simulink model "MotorControllerSimulation"  (R2016a)
settings: Solver=VariableStepAuto  StartTime=0.0  StopTime=simTime  RelTol=1e-3
values from neighbouring files (symbols this model uses):
  currentSensorResistance = 0.001    [Initialize.m]
  D_Current = 0    [Initialize.m]
  D_Velocity = 0    [Initialize.m]
  dampingCoefficient = 0    [Initialize.m]
  driverResistance = 1    [Initialize.m]
  gm = 1 / 0.0013    (= 769.230769231)    [Initialize.m]
  I_Current = 1    [Initialize.m]
  I_Velocity = 1    [Initialize.m]
  maxCurrent = 30    [Initialize.m]
  maxVelocity = 1000    [Initialize.m]
  mosfetGateResistance = 1    [Initialize.m]
  motorResistance = 1    [Initialize.m]
  P_Current = 1    [Initialize.m]
  P_Velocity = 1    [Initialize.m]
  sampleRate = 1000    [Initialize.m]
  switchingPeriod = 1/switchingFrequency    (= 0.0002)    [Initialize.m]
  targetVelocity = 300    [Initialize.m]
  torqueConstant = 1    [Initialize.m]
libraries: fl_lib x25, nesl_utility x5, simulink x4
settings Model: Creator=Koltin Kosik-Harvey  LastModifiedBy=Koltin Kosik-Harvey

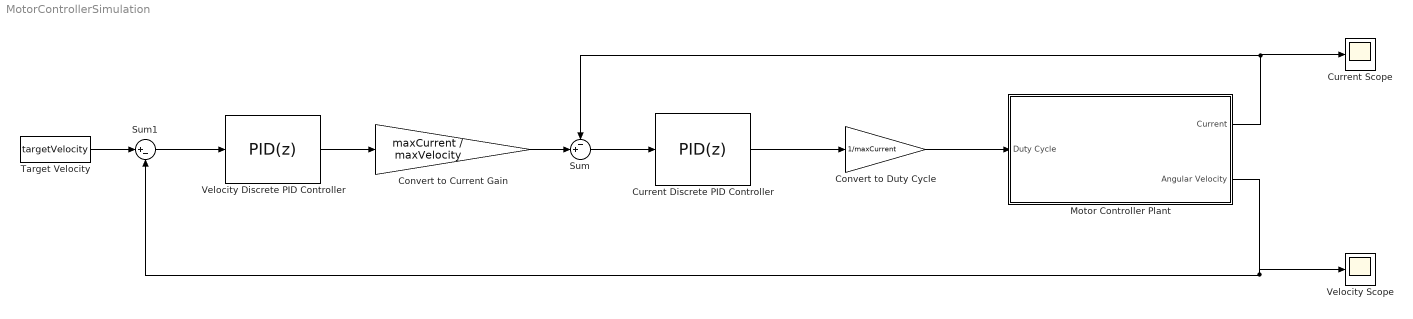
== system MotorControllerSimulation ==
  Convert to Current Gain : Gain  Gain=maxCurrent / maxVelocity
  Convert to Duty Cycle : Gain  Gain=1/maxCurrent
  Current Discrete PID Controller : simulink/Continuous/PID Controller  Controller=PID  TimeDomain=Discrete-time  SampleTime=sampleRate  IntegratorMethod=Forward Euler  FilterMethod=Forward Euler  Form=Parallel  UseFilter=on  ControllerParametersSource=internal  P=P_Current  I=I_Current  D=D_Current  N=100  InitialConditionSource=internal  InitialConditionForIntegrator=0  InitialConditionForFilter=0  ExternalReset=none  LimitOutput=on  UpperSaturationLimit=maxCurrent  LowerSaturationLimit=0  LinearizeAsGain=off  AntiWindupMode=none  Kb=1  TrackingMode=off  Kt=1  PParamMin=[]  PParamMax=[]  IParamMin=[]  IParamMax=[]  DParamMin=[]  DParamMax=[]  NParamMin=[]  NParamMax=[]  KbParamMin=[]  KbParamMax=[]  KtParamMin=[]  KtParamMax=[]  POutMin=[]  POutMax=[]  IOutMin=[]  IOutMax=[]  DOutMin=[]  DOutMax=[]  NOutMin=[]  NOutMax=[]  KbOutMin=[]  KbOutMax=[]  KtOutMin=[]  KtOutMax=[]  IntegratorOutMin=[]  IntegratorOutMax=[]  FilterOutMin=[]  FilterOutMax=[]  SumOutMin=[]  SumOutMax=[]  SumI1OutMin=[]  SumI1OutMax=[]  SumI2OutMin=[]  SumI2OutMax=[]  SumI3OutMin=[]  SumI3OutMax=[]  SumDOutMin=[]  SumDOutMax=[]  SaturationOutMin=[]  SaturationOutMax=[]  IntegratorContinuousStateAttributes=''  IntegratorStateMustResolveToSignalObject=off  IntegratorRTWStateStorageClass=Auto  FilterContinuousStateAttributes=''  FilterStateMustResolveToSignalObject=off  FilterRTWStateStorageClass=Auto  DifferentiatorICPrevScaledInput=0  DifferentiatorOutMin=[]  DifferentiatorOutMax=[]
  Current Scope : Scope
  Motor Controller Plant : Subsystem
  Sum : Sum  Inputs=-+|
  Sum1 : Sum  Inputs=|+-
  Target Velocity : Constant  Value=targetVelocity
  Velocity Discrete PID Controller : simulink/Continuous/PID Controller  Controller=PID  TimeDomain=Discrete-time  SampleTime=sampleRate  IntegratorMethod=Forward Euler  FilterMethod=Forward Euler  Form=Parallel  UseFilter=on  ControllerParametersSource=internal  P=P_Velocity  I=I_Velocity  D=D_Velocity  N=100  InitialConditionSource=internal  InitialConditionForIntegrator=0  InitialConditionForFilter=0  ExternalReset=none  LimitOutput=on  UpperSaturationLimit=maxVelocity  LowerSaturationLimit=0  LinearizeAsGain=off  AntiWindupMode=none  Kb=1  TrackingMode=off  Kt=1  PParamMin=[]  PParamMax=[]  IParamMin=[]  IParamMax=[]  DParamMin=[]  DParamMax=[]  NParamMin=[]  NParamMax=[]  KbParamMin=[]  KbParamMax=[]  KtParamMin=[]  KtParamMax=[]  POutMin=[]  POutMax=[]  IOutMin=[]  IOutMax=[]  DOutMin=[]  DOutMax=[]  NOutMin=[]  NOutMax=[]  KbOutMin=[]  KbOutMax=[]  KtOutMin=[]  KtOutMax=[]  IntegratorOutMin=[]  IntegratorOutMax=[]  FilterOutMin=[]  FilterOutMax=[]  SumOutMin=[]  SumOutMax=[]  SumI1OutMin=[]  SumI1OutMax=[]  SumI2OutMin=[]  SumI2OutMax=[]  SumI3OutMin=[]  SumI3OutMax=[]  SumDOutMin=[]  SumDOutMax=[]  SaturationOutMin=[]  SaturationOutMax=[]  IntegratorContinuousStateAttributes=''  IntegratorStateMustResolveToSignalObject=off  IntegratorRTWStateStorageClass=Auto  FilterContinuousStateAttributes=''  FilterStateMustResolveToSignalObject=off  FilterRTWStateStorageClass=Auto  DifferentiatorICPrevScaledInput=0  DifferentiatorOutMin=[]  DifferentiatorOutMax=[]
  Velocity Scope : Scope
  wires:
  Velocity Discrete PID Controller/1 -> Convert to Current Gain/1
  Current Discrete PID Controller/1 -> Convert to Duty Cycle/1
  Convert to Duty Cycle/1 -> Motor Controller Plant/1(Duty Cycle)
  Motor Controller Plant/1("Current ") -> Current Scope/1, Sum/1
  Convert to Current Gain/1 -> Sum/2
  Sum/1 -> Current Discrete PID Controller/1
  Motor Controller Plant/2(Angular Velocity) -> Sum1/2, Velocity Scope/1
  Target Velocity/1 -> Sum1/1
  Sum1/1 -> Velocity Discrete PID Controller/1

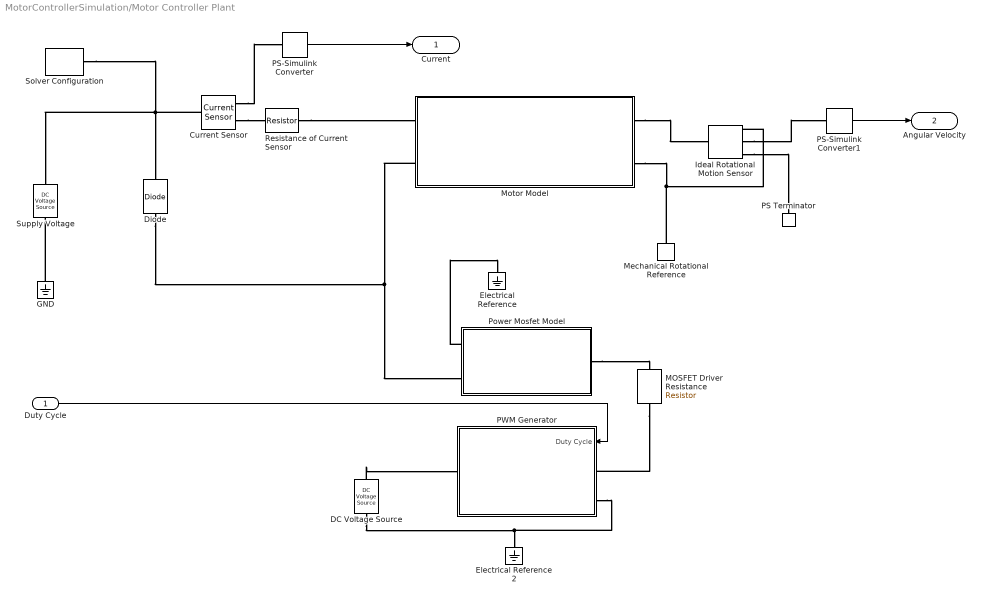
== system MotorControllerSimulation/Motor Controller Plant ==
  Duty Cycle : Inport
  Current Sensor : fl_lib/Electrical/Electrical Sensors/Current Sensor
  DC Voltage Source : fl_lib/Electrical/Electrical Sources/DC Voltage Source  v0=gateVoltage V
  Diode : fl_lib/Electrical/Electrical Elements/Diode  Vf=0.03 V  Ron=0.0001 Ohm  Goff=1e-8 1/Ohm  i_specify=off  i_priority=None  i=0 A  v_specify=off  v_priority=None  v=0 V
  Electrical Reference : fl_lib/Electrical/Electrical Elements/Electrical Reference
  Electrical Reference 2 : fl_lib/Electrical/Electrical Elements/Electrical Reference
  GND : fl_lib/Electrical/Electrical Elements/Electrical Reference
  Ideal Rotational Motion Sensor : fl_lib/Mechanical/Mechanical Sensors/Ideal Rotational Motion Sensor  offset=0 rad
  MOSFET Driver Resistance : fl_lib/Electrical/Electrical Elements/Resistor  R=driverResistance Ohm  i_specify=off  i_priority=None  i=0 A  v_specify=off  v_priority=None  v=0 V
  Mechanical Rotational Reference : fl_lib/Mechanical/Rotational Elements/Mechanical Rotational Reference
  Motor Model : Subsystem
  PS Terminator : fl_lib/Physical Signals/Sinks/PS Terminator
  PS-Simulink Converter : nesl_utility/PS-Simulink Converter  PhysicalDomain=network_engine_domain  SubClassName=ps_output  LeftPortType=input  RightPortType=output  PseudoPeriodic=off  Frequencies=[]  Unit=1  AffineConversion=off
  PS-Simulink Converter1 : nesl_utility/PS-Simulink Converter  PhysicalDomain=network_engine_domain  SubClassName=ps_output  LeftPortType=input  RightPortType=output  PseudoPeriodic=off  Frequencies=[]  Unit=1  AffineConversion=off
  PWM Generator : Subsystem
  Power Mosfet Model : Subsystem
  "Resistance of Current Sensor " : fl_lib/Electrical/Electrical Elements/Resistor  R=currentSensorResistance Ohm  i_specify=off  i_priority=None  i=0 A  v_specify=off  v_priority=None  v=0 V
  Solver Configuration : nesl_utility/Solver Configuration  PhysicalDomain=network_engine_domain  SubClassName=solver  LeftPortType=input  RightPortType=generic  Accelerate=off  Tones=[]  Harmonics=[]  SimulateNoise=off  Profile=off  UseLocalSampling=off  EnableSwitchedLinearOptims=on  FrequencyDomain=off  UseCCode=off  RelTol=0.001  AbsTol=1e-06  MinStep=1e-09  ToWorkspace=off  RevertToSquareIcSolve=off  NumHomotopyIterations=100  PhasorMode=off  PhasorModeNumHarmonics=1  OverrideAbsTol=off  DoDC=off  ResidualTolerance=1e-09  UseLocalSolver=off  LocalSolverChoice=NE_BACKWARD_EULER_ADVANCER  LocalSolverSampleTime=0.001  DoFixedCost=off  MaxNonlinIter=3  MaxModeIter=2  LinearAlgebra=Sparse  DelaysMemoryBudget=1024  AutomaticFiltering=on  FilteringTimeConstant=0.001
  Supply Voltage : fl_lib/Electrical/Electrical Sources/DC Voltage Source  v0=supplyVoltage V
  "Current " : Outport
  Angular Velocity : Outport  Port=2
  wires:
  Duty Cycle/1 -> PWM Generator/1(Duty Cycle)
  PS-Simulink Converter/1 -> "Current "/1
  PS-Simulink Converter1/1 -> Angular Velocity/1
  connections:
  DC Voltage Source/LConn1 -- PWM Generator/RConn1
  Power Mosfet Model/LConn1 -- MOSFET Driver Resistance/RConn1
  PWM Generator/LConn2 -- DC Voltage Source/RConn1 -- Electrical Reference 2/LConn1
  Current Sensor/RConn2 -- "Resistance of Current Sensor "/LConn1
  "Resistance of Current Sensor "/RConn1 -- Motor Model/LConn1
  Ideal Rotational Motion Sensor/RConn2 -- PS-Simulink Converter1/LConn1
  Power Mosfet Model/RConn1 -- Electrical Reference/LConn1
  Motor Model/RConn1 -- Ideal Rotational Motion Sensor/LConn1
  Current Sensor/RConn1 -- PS-Simulink Converter/LConn1
  Ideal Rotational Motion Sensor/RConn3 -- PS Terminator/LConn1
  Motor Model/LConn2 -- Diode/LConn1 -- Power Mosfet Model/RConn2
  Motor Model/RConn2 -- Ideal Rotational Motion Sensor/RConn1 -- Mechanical Rotational Reference/LConn1
  Current Sensor/LConn1 -- Solver Configuration/RConn1 -- Supply Voltage/LConn1 -- Diode/RConn1
  MOSFET Driver Resistance/LConn1 -- PWM Generator/LConn1
  GND/LConn1 -- Supply Voltage/RConn1

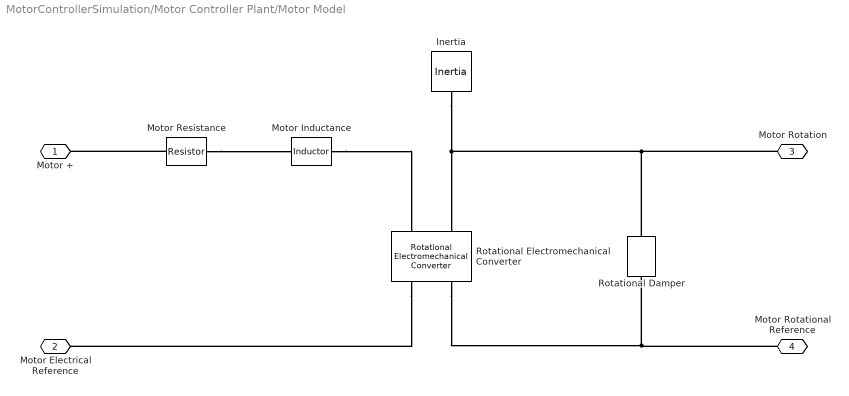
== system MotorControllerSimulation/Motor Controller Plant/Motor Model ==
  Inertia : fl_lib/Mechanical/Rotational Elements/Inertia  inertia=motorInertia kg*m^2  w_specify=off  w_priority=High  w=0 rad/s  t_specify=off  t_priority=None  t=0 N*m
  Motor Resistance : fl_lib/Electrical/Electrical Elements/Resistor  R=motorResistance Ohm  i_specify=off  i_priority=None  i=0 A  v_specify=off  v_priority=None  v=0 V
  Motor Inductance : fl_lib/Electrical/Electrical Elements/Inductor  l=motorInductance H  r=0 Ohm  g=1e-9 1/Ohm  i_specify=off  i_priority=None  i=0 A  v_specify=off  v_priority=None  v=0 V  i_L_specify=off  i_L_priority=High  i_L=0 A
  Rotational Electromechanical Converter : fl_lib/Electrical/Electrical Elements/Rotational Electromechanical Converter  K=torqueConstant V/(rad/s)  i_specify=off  i_priority=None  i=0 A  v_specify=off  v_priority=None  v=0 V  t_specify=off  t_priority=None  t=0 N*m  w_specify=off  w_priority=None  w=0 rad/s
  Rotational Damper : fl_lib/Mechanical/Rotational Elements/Rotational Damper  D=dampingCoefficient N*m/(rad/s)  w_specify=off  w_priority=None  w=0 rad/s  t_specify=off  t_priority=None  t=0 N*m
  Motor + : PMIOPort  Port=1  Side=Left
  Motor Electrical Reference : PMIOPort  Port=2  Side=Left
  Motor Rotation : PMIOPort  Port=3  Side=Right
  " Motor Rotational Reference" : PMIOPort  Port=4  Side=Right
  connections:
  Rotational Electromechanical Converter/RConn1 -- Motor Electrical Reference/RConn1
  Rotational Electromechanical Converter/RConn2 -- " Motor Rotational Reference"/RConn1 -- Rotational Damper/LConn1
  Motor Resistance/LConn1 -- Motor Inductance/RConn1
  Inertia/LConn1 -- Motor Rotation/RConn1 -- Rotational Damper/RConn1 -- Rotational Electromechanical Converter/LConn2
  Motor Inductance/LConn1 -- Rotational Electromechanical Converter/LConn1
  Motor Resistance/RConn1 -- Motor +/RConn1

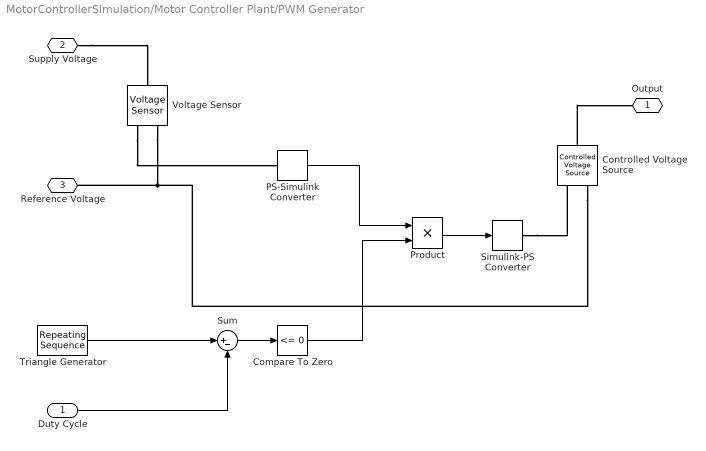
== system MotorControllerSimulation/Motor Controller Plant/PWM Generator ==
  Duty Cycle : Inport
  Compare To Zero : simulink/Logic and Bit Operations/Compare To Zero  relop=<=  OutDataTypeStr=boolean
  Controlled Voltage Source : fl_lib/Electrical/Electrical Sources/Controlled Voltage Source
  PS-Simulink Converter : nesl_utility/PS-Simulink Converter  PhysicalDomain=network_engine_domain  SubClassName=ps_output  LeftPortType=input  RightPortType=output  PseudoPeriodic=off  Frequencies=[]  Unit=1  AffineConversion=off
  Product : Product
  Simulink-PS Converter : nesl_utility/Simulink-PS Converter  PhysicalDomain=network_engine_domain  SubClassName=ps_input  LeftPortType=input  RightPortType=output  PseudoPeriodic=off  Frequencies=[]  NoiseDistribution=none  NoiseParameters=[]  Unit=1  AffineConversion=off  InputFiltering=off  SimscapeFilterOrder=1  InputFilterTimeConstant=0.001  UdotUserProvided=1
  Sum : Sum  Inputs=|+-
  Triangle Generator : simulink/Sources/Repeating Sequence  rep_seq_t=[0 switchingPeriod/2 switchingPeriod]  rep_seq_y=[0 1 0]
  Voltage Sensor : fl_lib/Electrical/Electrical Sensors/Voltage Sensor
  Output : PMIOPort  Port=1  Side=Left
  Supply Voltage : PMIOPort  Port=2  Side=Right
  Reference Voltage : PMIOPort  Port=3  Side=Left
  wires:
  Duty Cycle/1 -> Sum/2
  Triangle Generator/1 -> Sum/1
  Sum/1 -> Compare To Zero/1
  Compare To Zero/1 -> Product/2
  PS-Simulink Converter/1 -> Product/1
  Product/1 -> Simulink-PS Converter/1
  connections:
  Supply Voltage/RConn1 -- Voltage Sensor/LConn1
  Voltage Sensor/RConn2 -- Reference Voltage/RConn1 -- Controlled Voltage Source/RConn2
  Voltage Sensor/RConn1 -- PS-Simulink Converter/LConn1
  Controlled Voltage Source/LConn1 -- Output/RConn1
  Simulink-PS Converter/RConn1 -- Controlled Voltage Source/RConn1

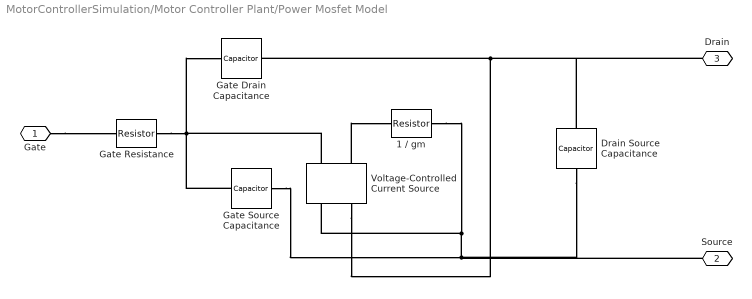
== system MotorControllerSimulation/Motor Controller Plant/Power Mosfet Model ==
  1 / gm : fl_lib/Electrical/Electrical Elements/Resistor  R=1 / gm Ohm  i_specify=off  i_priority=None  i=0 A  v_specify=off  v_priority=None  v=0 V
  Drain Source Capacitance : fl_lib/Electrical/Electrical Elements/Capacitor  c=drainSourceCapacitance F  r=1e-6 Ohm  g=0 1/Ohm  i_specify=off  i_priority=None  i=0 A  v_specify=off  v_priority=None  v=0 V  vc_specify=off  vc_priority=High  vc=0 V
  Gate Resistance : fl_lib/Electrical/Electrical Elements/Resistor  R=mosfetGateResistance Ohm  i_specify=off  i_priority=None  i=0 A  v_specify=off  v_priority=None  v=0 V
  Gate Drain Capacitance : fl_lib/Electrical/Electrical Elements/Capacitor  c=gateDrainCapacitance F  r=1e-6 Ohm  g=0 1/Ohm  i_specify=off  i_priority=None  i=0 A  v_specify=off  v_priority=None  v=0 V  vc_specify=off  vc_priority=High  vc=0 V
  "Gate Source Capacitance " : fl_lib/Electrical/Electrical Elements/Capacitor  c=gateSourceCapacitance F  r=1e-6 Ohm  g=0 1/Ohm  i_specify=off  i_priority=None  i=0 A  v_specify=off  v_priority=None  v=0 V  vc_specify=off  vc_priority=High  vc=0 V
  Voltage-Controlled Current Source : fl_lib/Electrical/Electrical Sources/Voltage-Controlled Current Source  K=1 1/Ohm  v1_specify=off  v1_priority=None  v1=0 V  i2_specify=off  i2_priority=None  i2=0 A
  "Gate " : PMIOPort  Port=1  Side=Left
  " Source" : PMIOPort  Port=2  Side=Right
  " Drain" : PMIOPort  Port=3  Side=Right
  connections:
  Gate Resistance/RConn1 -- Voltage-Controlled Current Source/LConn1 -- "Gate Source Capacitance "/LConn1 -- Gate Drain Capacitance/LConn1
  Voltage-Controlled Current Source/LConn2 -- 1 / gm/LConn1
  "Gate Source Capacitance "/RConn1 -- " Source"/RConn1 -- Drain Source Capacitance/LConn1 -- 1 / gm/RConn1 -- Voltage-Controlled Current Source/RConn1
  "Gate "/RConn1 -- Gate Resistance/LConn1
  Voltage-Controlled Current Source/RConn2 -- " Drain"/RConn1 -- Drain Source Capacitance/RConn1 -- Gate Drain Capacitance/RConn1
